simulink model "Tape_motion_dynamic_ideal"  (R2017b)
settings: Solver=VariableStepAuto  StartTime=0.0  StopTime=runtime  RelTol=1e-3
values from neighbouring files (symbols this model uses):
  C = tf([0.5 2.5],[1 2 0])    [script_2nd_order.m]
  Ts = 0.4    [script_2nd_order.m]    (also in script_new_model.m = 0.00833333333333)
undefined symbols (not defined in the file or in its folder): A, A1, B, B1, C1, D, D1, K, step_final, step_init, step_time, tau
libraries: dspsigops x4
settings Model: Creator=e25756  LastModifiedBy=e25756

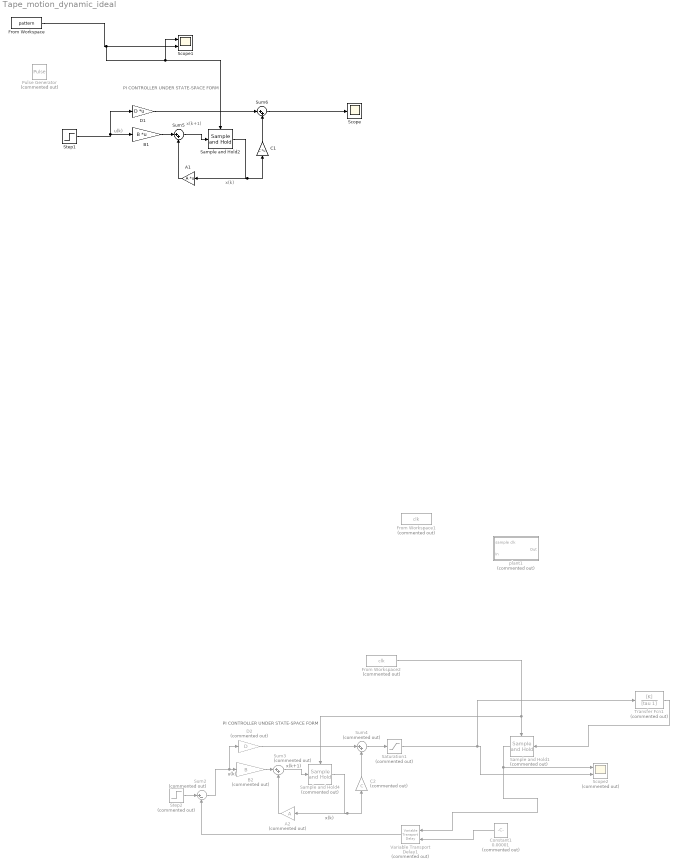
== system Tape_motion_dynamic_ideal ==
  note: x(k)
  note: u(k)
  note: x(k+1)
  note: PI CONTROLLER UNDER STATE-SPACE FORM
  note: u(k)
  note: x(k)
  note: x(k+1)
  note: PI CONTROLLER UNDER STATE-SPACE FORM
  A1 : Gain  Gain=A  Multiplication=Matrix(K*u)
  A2 : Gain  Commented=on  Gain=A
  B1 : Gain  Gain=B  Multiplication=Matrix(K*u)
  B2 : Gain  Commented=on  Gain=B
  C1 : Gain  Gain=C  Multiplication=Matrix(K*u)
  C2 : Gain  Commented=on  Gain=C
  Constant1 : Constant  Commented=on  Value=0.00001
  D1 : Gain  Gain=D  Multiplication=Matrix(K*u)
  D2 : Gain  Commented=on  Gain=D
  From Workspace : FromWorkspace  VariableName=pattern  SampleTime=Ts*0.1  Interpolate=off  OutputAfterFinalValue=Holding final value
  From Workspace1 : FromWorkspace  Commented=on  VariableName=clk  SampleTime=0.0001  Interpolate=off  OutputAfterFinalValue=Setting to zero
  From Workspace2 : FromWorkspace  Commented=on  VariableName=clk  SampleTime=0
  Pulse Generator : DiscretePulseGenerator  Commented=on  PulseType=Time based  Period=Ts  PulseWidth=50
  Sample and Hold1 : dspsigops/Sample and Hold  Commented=on  trig=Rising edge  initCond=0  latchinput=on
  Sample and Hold2 : dspsigops/Sample and Hold  trig=Rising edge  initCond=0  latchinput=on
  Sample and Hold4 : dspsigops/Sample and Hold  Commented=on  trig=Rising edge  initCond=0  latchinput=on
  Saturation1 : Saturate  Commented=on  UpperLimit=5  LowerLimit=0
  Scope : Scope
  Scope1 : Scope  NumInputPorts=2
  Scope2 : Scope  Commented=on  NumInputPorts=2
  Step1 : Step  Time=0  SampleTime=Ts*0.1
  Step2 : Step  Commented=on  Time=step_time  Before=step_init  After=step_final  SampleTime=Ts
  Sum2 : Sum  Commented=on  Inputs=|+-
  Sum3 : Sum  Commented=on  Inputs=|++
  Sum4 : Sum  Commented=on  Inputs=|++
  Sum5 : Sum  Inputs=|++
  Sum6 : Sum  Inputs=|++
  Transfer Fcn1 : TransferFcn  Commented=on  Numerator=[K]  Denominator=[tau 1]
  Variable Transport Delay1 : VariableTransportDelay  Commented=on  VariableDelayType=Variable transport delay  MaximumDelay=0.01
  plant1 : Subsystem  Commented=on
  wires:
  Step1/1 -> D1/1, B1/1
  B1/1 -> Sum5/1
  A1/1 -> Sum5/2
  D1/1 -> Sum6/1
  Sample and Hold2/1 -> C1/1, A1/1
  C1/1 -> Sum6/2
  Sum5/1 -> Sample and Hold2/1
  Sum6/1 -> Scope/1
  B2/1 -> Sum3/1
  Step2/1 -> Sum2/1
  Sum2/1 -> D2/1, B2/1
  A2/1 -> Sum3/2
  C2/1 -> Sum4/2
  Sum3/1 -> Sample and Hold4/1
  Sum4/1 -> Saturation1/1
  D2/1 -> Sum4/1
  Sample and Hold4/1 -> C2/1, A2/1
  Variable Transport Delay1/1 -> Sum2/2
  Saturation1/1 -> Transfer Fcn1/1, Scope2/2
  Transfer Fcn1/1 -> Sample and Hold1/1
  From Workspace2/1 -> Sample and Hold4/Trigger, Sample and Hold1/Trigger
  Sample and Hold1/1 -> Scope2/1, Variable Transport Delay1/1
  Constant1/1 -> Variable Transport Delay1/2
  From Workspace/1 -> Scope1/1, Sample and Hold2/Trigger, Scope1/2

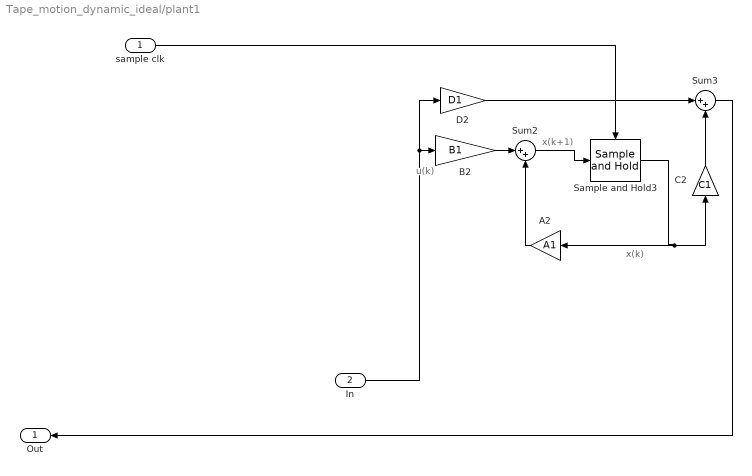
== system Tape_motion_dynamic_ideal/plant1 ==
  note: x(k)
  note: u(k)
  note: x(k+1)
  sample clk : Inport
  In : Inport  Port=2
  A2 : Gain  Gain=A1
  B2 : Gain  Gain=B1
  C2 : Gain  Gain=C1
  D2 : Gain  Gain=D1
  Sample and Hold3 : dspsigops/Sample and Hold  trig=Rising edge  initCond=0  latchinput=on
  Sum2 : Sum  Inputs=|++
  Sum3 : Sum  Inputs=|++
  Out : Outport
  wires:
  Sum3/1 -> Out/1
  Sum2/1 -> Sample and Hold3/1
  A2/1 -> Sum2/2
  C2/1 -> Sum3/2
  D2/1 -> Sum3/1
  Sample and Hold3/1 -> C2/1, A2/1
  B2/1 -> Sum2/1
  In/1 -> D2/1, B2/1
  sample clk/1 -> Sample and Hold3/Trigger
